simulink model "quadrotor_adaptive_control"  (R2025b)
settings: Solver=ode4  StartTime=0.0  StopTime=150  FixedStep=0.001  MaxStep=1e-3  RelTol=1e-6
values from neighbouring files (symbols this model uses):
  pi_hat0 = [0.899; 0.009; 0.009; 0.015]    [pi_hat_init.m]
undefined symbols (not defined in the file or in its folder): F, Light, MIL
libraries: simulink x5, aerolibwind2 x3
(part 2 of 2)

== matlab function quadrotor_adaptive_control/Adaptive Control + disturbance estimator controller for Quadrotor Model/Quadrotor adaptive plant/disturbance_adder ==
  data: dState input; V_wind input; w_wind input; dState_fin output size=12
function dState_fin = disturbance_adder(dState, V_wind, w_wind)
    % 1. NOMINAL dState UNPACKING
    dx0 = dState(1); dy0 = dState(2); dz0 = dState(3); % Velocità lineari
    du0 = dState(4); dv0 = dState(5); dw0 = dState(6); % Accelerazioni lineari
    dphi0 = dState(7); dtheta0 = dState(8); dpsi0 = dState(9); % Velocità angolari
    dp0 = dState(10); dq0 = dState(11); dr0 = dState(12); % Accelerazioni angolari
    
    % 2. V_wind and w_wind UNPACKING
    V_wind_x = V_wind(1); V_wind_y = V_wind(2); V_wind_z = V_wind(3);
    w_wind_phi = w_wind(1); w_wind_theta = w_wind(2); w_wind_psi = w_wind(3);
    
    % 3. Drag coefficients 
    Kd_lin = 0.6;  
    Kd_ang = 0.5;  
    
    % 4. Drag wind accelerations
    a_wind_x = Kd_lin * (V_wind_x - dx0);
    a_wind_y = Kd_lin * (V_wind_y - dy0);
    a_wind_z = Kd_lin * (V_wind_z - dz0);
    
    alpha_wind_phi = Kd_ang * (w_wind_phi - dphi0);
    alpha_wind_theta = Kd_ang * (w_wind_theta - dtheta0);
    alpha_wind_psi = Kd_ang * (w_wind_psi - dpsi0);
    
    % 5. Injenction of disturbance (on acceleration)
    du_fin = du0 + a_wind_x;
    dv_fin = dv0 + a_wind_y;
    dw_fin = dw0 + a_wind_z;
    
    dp_fin = dp0 + alpha_wind_phi;
    dq_fin = dq0 + alpha_wind_theta;
    dr_fin = dr0 + alpha_wind_psi;
    
    % 6. PACKING FINAL dState
    dState_fin = [dx0; dy0; dz0; du_fin; dv_fin; dw_fin; dphi0; dtheta0; dpsi0; dp_fin; dq_fin; dr_fin];
 
end

== matlab function quadrotor_adaptive_control/Adaptive Controller for Quadrotor Model/Quadrotor adaptive plant/Motor_losses/Motor_loss ==
  data: Tau_real output; Tau_ideal input; f1_step input; f2_step input; f3_step input; f4_step input
function Tau_real = Motor_Variation(Tau_ideal, f1_step, f2_step, f3_step, f4_step)
    % f1_step_1: 0 se il motore è rotto, 1 se è sano
    
    % Parametri geometrici
    l = 0.072; c = 0.015;
    
    % Definizione matrice di MIXING
    M = [ 1,  1,  1,  1;
          0,  l,  0, -l;
         -l,  0,  l,  0;
          c, -c,  c, -c];
    
    % Extraction of f1, essendo     Tau_ideal = M * f 
    M_inv = inv(M);
    f1_ideal = M_inv(1,:) * Tau_ideal; 
    f2_ideal = M_inv(2,:) * Tau_ideal; 
    f3_ideal = M_inv(3,:) * Tau_ideal; 
    f4_ideal = M_inv(4,:) * Tau_ideal; 

    perdita_f1 = f1_ideal * f1_step;
    perdita_f2 = f2_ideal * f2_step;
    perdita_f3 = f3_ideal * f3_step;
    perdita_f4 = f4_ideal * f4_step;
    
    % 3. Traduco l'impatto della perdita sul vettore Tau 
    impatto_su_Tau = M(:,1) * perdita_f1;
    impatto_su_Tau1 = M(:,2) * perdita_f2;
    impatto_su_Tau2 = M(:,3) * perdita_f3;
    impatto_su_Tau3 = M(:,4) * perdita_f4;

    % 4. Sottraiamo il fattore di perdita del tau "totale" dal tau reale
    % Tau_real = Tau_ideal - impatto_su_Tau;
    % Tau_real = Tau_real - impatto_su_Tau1;
    % Tau_real = Tau_real - impatto_su_Tau2;
    % Tau_real = Tau_real - impatto_su_Tau3;


    Tau_real = Tau_ideal - (impatto_su_Tau+impatto_su_Tau1+impatto_su_Tau2+impatto_su_Tau3);
end

== matlab function quadrotor_adaptive_control/Adaptive Control + disturbance estimator controller for Quadrotor Model/Quadrotor adaptive plant/Motor_losses/Motor_loss ==
  data: Tau_real output; Tau_ideal input; f1_step input; f2_step input; f3_step input; f4_step input
function Tau_real = Motor_Variation(Tau_ideal, f1_step, f2_step, f3_step, f4_step)
    % f1_step_1: 0 se il motore è rotto, 1 se è sano
    
    % Parametri geometrici
    l = 0.072; c = 0.015;
    
    % Definizione matrice di MIXING
    M = [ 1,  1,  1,  1;
          0,  l,  0, -l;
         -l,  0,  l,  0;
          c, -c,  c, -c];
    
    % Extraction of f1, essendo     Tau_ideal = M * f 
    M_inv = inv(M);
    f1_ideal = M_inv(1,:) * Tau_ideal; 
    f2_ideal = M_inv(2,:) * Tau_ideal; 
    f3_ideal = M_inv(3,:) * Tau_ideal; 
    f4_ideal = M_inv(4,:) * Tau_ideal; 

    perdita_f1 = f1_ideal * f1_step;
    perdita_f2 = f2_ideal * f2_step;
    perdita_f3 = f3_ideal * f3_step;
    perdita_f4 = f4_ideal * f4_step;
    
    % 3. Traduco l'impatto della perdita sul vettore Tau 
    impatto_su_Tau = M(:,1) * perdita_f1;
    impatto_su_Tau1 = M(:,2) * perdita_f2;
    impatto_su_Tau2 = M(:,3) * perdita_f3;
    impatto_su_Tau3 = M(:,4) * perdita_f4;

    % 4. Sottraiamo il fattore di perdita del tau "totale" dal tau reale
    % Tau_real = Tau_ideal - impatto_su_Tau;
    % Tau_real = Tau_real - impatto_su_Tau1;
    % Tau_real = Tau_real - impatto_su_Tau2;
    % Tau_real = Tau_real - impatto_su_Tau3;


    Tau_real = Tau_ideal - (impatto_su_Tau+impatto_su_Tau1+impatto_su_Tau2+impatto_su_Tau3);
end

== matlab function quadrotor_adaptive_control/Linearized Quadrotor Model with PD controller/Quad PD Plant/Motor_losses/Motor_loss ==
  data: Tau_real output; Tau_ideal input; f1_step input; f2_step input; f3_step input; f4_step input
function Tau_real = Motor_Variation(Tau_ideal, f1_step, f2_step, f3_step, f4_step)
    % f1_step_1: 0 se il motore è rotto, 1 se è sano
    
    % Parametri geometrici
    l = 0.072; c = 0.015;
    
    % Definizione matrice di MIXING
    M = [ 1,  1,  1,  1;
          0,  l,  0, -l;
         -l,  0,  l,  0;
          c, -c,  c, -c];
    
    % Extraction of f1, essendo     Tau_ideal = M * f 
    M_inv = inv(M);
    f1_ideal = M_inv(1,:) * Tau_ideal; 
    f2_ideal = M_inv(2,:) * Tau_ideal; 
    f3_ideal = M_inv(3,:) * Tau_ideal; 
    f4_ideal = M_inv(4,:) * Tau_ideal; 

    perdita_f1 = f1_ideal * f1_step;
    perdita_f2 = f2_ideal * f2_step;
    perdita_f3 = f3_ideal * f3_step;
    perdita_f4 = f4_ideal * f4_step;
    
    % 3. Traduco l'impatto della perdita sul vettore Tau 
    impatto_su_Tau = M(:,1) * perdita_f1;
    impatto_su_Tau1 = M(:,2) * perdita_f2;
    impatto_su_Tau2 = M(:,3) * perdita_f3;
    impatto_su_Tau3 = M(:,4) * perdita_f4;

    % 4. Sottraiamo il fattore di perdita del tau "totale" dal tau reale
    % Tau_real = Tau_ideal - impatto_su_Tau;
    % Tau_real = Tau_real - impatto_su_Tau1;
    % Tau_real = Tau_real - impatto_su_Tau2;
    % Tau_real = Tau_real - impatto_su_Tau3;


    Tau_real = Tau_ideal - (impatto_su_Tau+impatto_su_Tau1+impatto_su_Tau2+impatto_su_Tau3);
end

== matlab function quadrotor_adaptive_control/Adaptive Control + disturbance estimator controller for Quadrotor Model/Wind extractor/MATLAB Function ==
  data: dState input; f_wnoise output; State input
function f_wnoise = selector(dState, State)

    m0 = 0.899;
    g  = 9.81;

    du = dState(4);
    dv = dState(5);
    dw = dState(6);

    phi   = State(7);
    theta = State(8);
    psi   = State(9);

    cphi = cos(phi);
    cth  = cos(theta);

    den = cphi * cth;
    %just a way to rebuild thrust in quadrotor's frame body coordinates and not world's
   
    if abs(den) < 0.2
        den = sign(den) * 0.2;
    end

    F_total = m0 * (dw + g) / den; %getting just the motors' thrust using its z-axis direction OF QUADROTOR!!!

  % We estimate the total rotor thrust from the vertical (world-z) dynamics.
% Assuming wind has negligible component along world-z, the z channel is
% relatively clean compared to x-y channels.
%
% The rotor thrust acts along the quadrotor body z-axis, not along world-z
% unless the vehicle is level (hover condition). Therefore, its vertical
% component in world coordinates is:
%
%   Fz = F_total * cos(phi) * cos(theta)
%
% Using the z dynamics, we reconstruct F_total, then project it onto the
% world x and y axes. This gives an estimate of the lateral acceleration
% caused only by thrust, so the remaining x-y residual can be attributed
% mainly to wind/disturbances.
%
% Important: even if this thrust has been generated by the controller to
% counteract wind, it is still rotor thrust, not wind itself. In other
% words, it represents the plant control action in the lateral channels.
% The wind estimate is obtained only as the residual:
%
%   wind_xy = m*a_xy - thrust_xy
%
% so thrust_xy is the modeled lateral contribution due to control, while
% the remaining unexplained part is attributed to external disturbances.
% This is possible because wind is not instrinsic to quadrotor plant dynamics.


    F_x = (sin(theta)*cos(psi) + sin(phi)*cos(theta)*sin(psi)) * F_total;
    F_y = (sin(theta)*sin(psi) - sin(phi)*cos(theta)*cos(psi)) * F_total;
    
    %if no wind is present it should go to zero (refer to the explainaition above.
    f_wnoise = m0*[du; dv] - [F_x; F_y];
end

== matlab function quadrotor_adaptive_control/Adaptive Controller for Quadrotor Model/Quadrotor adaptive plant/adaptive control dynamics ==
  data: State input; dState output; A input; m input; Ixx input; Iyy input; Izz input; z output; vel_mod output; rot_angles output
function [dState, z, vel_mod, rot_angles] = adp_dynamics(State, A, m, Ixx, Iyy, Izz)
    % 1. STATE EXTRACTION
    x = State(1); y = State(2); z = State(3); 
    u = State(4); v = State(5); w = State(6); 
    phi = State(7); theta = State(8); psi = State(9); 
    p = State(10); q = State(11); r = State(12);
    
    % 2. CONTROL INPUT EXTRACTION (Total thrust and body torques)
    F = A(1); 
    tau_phi = A(2); tau_theta = A(3); tau_psi = A(4);
    
    g = 9.81;
    
    % Mass-normalized thrust (Specific force)
    f_norm = F / m; 
    
    % Definition of trigonometric functions for computational semplicity
    c_phi = cos(phi); s_phi = sin(phi); t_phi = tan(phi);
    c_theta = cos(theta); s_theta = sin(theta); 
    c_psi = cos(psi); s_psi = sin(psi);
    
    % Linear kinematics (Translational velocities)
    dx = u; dy = v; dz = w;
    
    % Translational dynamics (Linear accelerations using Z-X-Y convention)
    du = (s_theta * c_psi + s_phi * c_theta * s_psi) * f_norm;
    dv = (s_theta * s_psi - s_phi * c_theta * c_psi) * f_norm;
    dw = (c_phi * c_theta) * f_norm - g;
    
    % Angular kinematics 
    % Note: Derived for the Z-X-Y rotation sequence
    dphi = c_theta * p + s_theta * r;
    dtheta = t_phi * s_theta * p + q - t_phi * c_theta * r;
    dpsi = -(s_theta / c_phi) * p + (c_theta / c_phi) * r;
    
    % Angular dynamics (Euler's equations of motion for a rigid body)
    dp = (tau_phi - (Izz - Iyy) * q * r) / Ixx;
    dq = (tau_theta - (Ixx - Izz) * p * r) / Iyy;
    dr = (tau_psi - (Iyy - Ixx) * p * q) / Izz;
    
    % Vector assembly (State derivative packing)
    dState = [dx; dy; dz; du; dv; dw; dphi; dtheta; dpsi; dp; dq; dr];

    %modulus of speed
    vel_mod = sqrt(v^2+u^2+w^2)+ 0.01;

    %rotational angles packing
    rot_angles = [phi, theta, psi];

end

== matlab function quadrotor_adaptive_control/Adaptive Controller for Quadrotor Model/Adaptive Controller/Adaptive controller ==
  data: State input; tau_vec output size=[4 1]; pi_hat input; Xd input; Yd input; Zd input; dpi_hat output size=4; dPsi_c input; dPhi_c input; phi_c output size=1; theta_c output size=1; dTheta_c input; psi_c output
function [tau_vec, dpi_hat, phi_c, theta_c, psi_c] = controller_adaptive( ...
    State, pi_hat, Xd, Yd, Zd, dPsi_c, dPhi_c, dTheta_c)

    % ============================================================
    % ADAPTIVE CONTROLLER (NO WIND COMPENSATION)
    % ============================================================

    % ---------- Tunable gains ----------
    Kd     = diag([2.0, 0.08, 0.08, 0.040]);
    Ks     = diag([5, 3.5, 3.5, 2]);
    Lambda = diag([5.0, 8.0, 8.0, 5.0]);
    Kpi    = diag([1.5, 0.003, 0.003, 0.008]);
    
    % leakage factcors
    sigma_pi = diag([0.20, 0.002, 0.002, 0.004]);

    % nominal parameters
    m0     = 0.899;
    Ixx0   = 0.009;
    Iyy0   = 0.009;
    Izz0   = 0.015;
    pi_nom = [m0; Ixx0; Iyy0; Izz0];

    g = 9.81;

    % practical quasi-hovering saturations
    % 
    % phi_max   = 0.35;  % [rad]    
    % theta_max = 0.35;    

    % ---------- 1) State extraction ----------
    x = State(1);   y = State(2);   z = State(3);
    u = State(4);   v = State(5);   w = State(6);
    phi = State(7); theta = State(8); psi = State(9);
    p = State(10);  q_rot = State(11); r = State(12);

    % ---------- 2) Desired references ----------
    x_d   = Xd(1);  dx_d   = Xd(2);  ddx_d   = Xd(3);
    y_d   = Yd(1);  dy_d   = Yd(2);  ddy_d   = Yd(3);
    z_d   = Zd(1);  dz_d   = Zd(2);  ddz_d   = Zd(3);

    % yaw fixed
    psi_d   = 0.0;
    dpsi_d  = 0.0;
    ddpsi_d = 0.0;

    % ---------- 3) Outer loop X-Y ----------
    e_x  = x - x_d;
    de_x = u - dx_d;

    e_y  = y - y_d;
    de_y = v - dy_d;

    % nominal desired accelerations (no wind compensation)
    a_x = ddx_d - 8.0*de_x - 15.0*e_x;
    a_y = ddy_d - 8.0*de_y - 15.0*e_y;


    % ---------- 4) Kinematic inversion ----------

    phi_c   = (1/g) * (a_x * sin(psi_d) - a_y * cos(psi_d));
    theta_c = (1/g) * (a_x * cos(psi_d) + a_y * sin(psi_d));
    psi_c   = psi_d;

    % done externally
    % phi_c   = min(max(phi_c,   -phi_max),   phi_max);
    % theta_c = min(max(theta_c, -theta_max), theta_max);

    % ---------- 5) Reference derivatives ----------
    dphi_c   = dPhi_c(1);
    ddphi_c  = dPhi_c(2);

    dtheta_c  = dTheta_c(1);
    ddtheta_c = dTheta_c(2);

    % dPsi_c currently unused

    % ---------- 6) Inner loop ----------
    e_z      = z - z_d;
    de_z     = w - dz_d;

    e_phi    = phi - phi_c;
    de_phi   = p - dphi_c;

    e_theta  = theta - theta_c;
    de_theta = q_rot - dtheta_c;

    e_psi    = psi - psi_d;
    de_psi   = r - dpsi_d;

    e_vec  = [e_z; e_phi; e_theta; e_psi];
    de_vec = [de_z; de_phi; de_theta; de_psi];
    ddq_d  = [ddz_d; ddphi_c; ddtheta_c; ddpsi_d];

    % sliding surface
    s = de_vec + Lambda * e_vec;

    % reference model
    dq_ref  = [dz_d; dphi_c; dtheta_c; dpsi_d] - Lambda * e_vec;
    ddq_ref = ddq_d - Lambda * de_vec;

    %p_ref  = dq_ref(2);
    q_ref  = dq_ref(3);
    r_ref  = dq_ref(4);

    dp_ref     = ddq_ref(2);
    dq_ref_att = ddq_ref(3);
    dr_ref     = ddq_ref(4);

    ddz_ref = ddq_ref(1);

    % ---------- 7) Regressor ----------
    Y_z = ddz_ref + g;

    Y_att = [ dp_ref,      -q_rot*r_ref,   q_rot*r_ref;
              p*r_ref,      dq_ref_att,   -p*r_ref;
             -p*q_ref,      p*q_ref,       dr_ref ];

    Y = blkdiag(Y_z, Y_att);

    % ---------- 8) Control law ----------
    tau_vec = Y*pi_hat - Kd*e_vec - Ks*s;

    % ---------- 9) Adaptive law ----------
    s_norm = norm(s);

    if s_norm > 0.02 %dead zone, no upper bound 
        dpi_hat = -Kpi * (Y.' * s) - sigma_pi * (pi_hat - pi_nom);
    else
        dpi_hat = -sigma_pi * (pi_hat - pi_nom);
    end
end

== matlab function quadrotor_adaptive_control/Adaptive Controller for Quadrotor Model/MATLAB Function1 ==
  data: State input; e_pos output; Xd input; Yd input; Zd input; de_pos output
function [e_pos, de_pos] = error_calculator(State, Xd, Yd, Zd)
    
    % --- 1. STATE EXTRACTION ---
  
    x = State(1); y = State(2); z = State(3);
    u = State(4); v = State(5); w = State(6);
    
    phi = State(7); theta = State(8); psi = State(9);
    p = State(10); q = State(11); r = State(12);

    % --- 2. OUTER LOOP ERRORS
    % Standard convention: Error = Actual - Desired
    e_x = x - Xd(1); de_x = u - Xd(2);
    e_y = y - Yd(1); de_y = v - Yd(2);
    e_z = z - Zd(1); de_z = w - Zd(2);
    
    e_pos = [e_x; e_y; e_z];
    de_pos = [de_x; de_y; de_z];
end

== matlab function quadrotor_adaptive_control/Linearized Quadrotor Model with PD controller/Quad PD Plant/PD model dynamics ==
  data: State input; dState output; tau input; m input; Ixx input; Iyy input; Izz input; z output; vel_mod output; rot_angles output
function [dState, z, vel_mod, rot_angles] = lin_dynamics(State, tau, m, Ixx, Iyy, Izz)
    
    % unpacking of state
    x = State(1); y = State(2); z = State(3); 
    u = State(4); v = State(5); w = State(6); 
    phi = State(7); theta = State(8); psi = State(9); 
    p = State(10); q = State(11); r = State(12);
    deltaF = tau(1);
    tau_phi = tau(2); tau_theta = tau(3); tau_psi = tau(4);
    
    g = 9.81;
    psi_bar = 0;
     
    dv_and_du = g * ...
        [sin(psi_bar), cos(psi_bar); -cos(psi_bar), sin(psi_bar)] * ...
        [phi; theta];
    
    % packed dynamics
    dState = [u; v; w; ...
        dv_and_du; (deltaF) / m;...
        p; q; r; ...
        tau_phi / Ixx; tau_theta / Iyy; tau_psi / Izz];
    
    %modulus of speed
    vel_mod = sqrt(v^2+u^2+w^2) + 0.01;
    
    
    %rotational angles packing
    rot_angles = [phi, theta, psi];
    
    
end

== matlab function quadrotor_adaptive_control/Adaptive Controller for Quadrotor Model/Quadrotor adaptive plant/disturbance_adder ==
  data: dState input; V_wind input; w_wind input; dState_fin output size=12
function dState_fin = disturbance_adder(dState, V_wind, w_wind)
    % 1. NOMINAL dState UNPACKING
    dx0 = dState(1); dy0 = dState(2); dz0 = dState(3); % Velocità lineari
    du0 = dState(4); dv0 = dState(5); dw0 = dState(6); % Accelerazioni lineari
    dphi0 = dState(7); dtheta0 = dState(8); dpsi0 = dState(9); % Velocità angolari
    dp0 = dState(10); dq0 = dState(11); dr0 = dState(12); % Accelerazioni angolari
    
    % 2. V_wind and w_wind UNPACKING
    V_wind_x = V_wind(1); V_wind_y = V_wind(2); V_wind_z = V_wind(3);
    w_wind_phi = w_wind(1); w_wind_theta = w_wind(2); w_wind_psi = w_wind(3);
    
    % 3. Drag coefficients 
     Kd_lin = 0.6;  
     Kd_ang = 0.5; 
    
    % 4. Drag wind accelerations
    a_wind_x = Kd_lin * (V_wind_x - dx0);
    a_wind_y = Kd_lin * (V_wind_y - dy0);
    a_wind_z = Kd_lin * (V_wind_z - dz0);
    
    alpha_wind_phi = Kd_ang * (w_wind_phi - dphi0);
    alpha_wind_theta = Kd_ang * (w_wind_theta - dtheta0);
    alpha_wind_psi = Kd_ang * (w_wind_psi - dpsi0);
    
    % 5. Injenction of disturbance (on acceleration)
    du_fin = du0 + a_wind_x;
    dv_fin = dv0 + a_wind_y;
    dw_fin = dw0 + a_wind_z;
    
    dp_fin = dp0 + alpha_wind_phi;
    dq_fin = dq0 + alpha_wind_theta;
    dr_fin = dr0 + alpha_wind_psi;
    
    % 6. PACKING FINAL dState
    dState_fin = [dx0; dy0; dz0; du_fin; dv_fin; dw_fin; dphi0; dtheta0; dpsi0; dp_fin; dq_fin; dr_fin];
 
end
